simulink model "untitled1"  (R2012b)
settings: Solver=ode45  StartTime=0.0  StopTime=10.0  RelTol=1e-9
settings Model: Creator=Katarina  LastModifiedBy=Katarina
settings DataIOCC: LimitDataPoints=off
settings DebuggingCC: SolverPrmCheckMsg=none

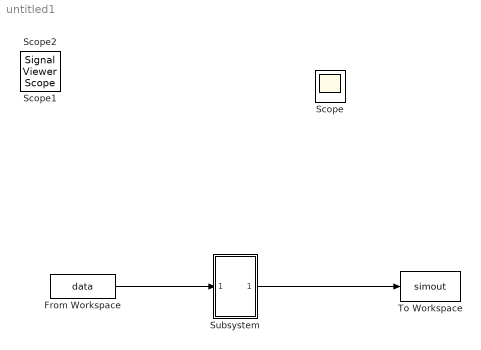
== system untitled1 ==
  From Workspace : FromWorkspace  VariableName=data  SampleTime=0
  Scope : Scope
  Subsystem : Subsystem
  To Workspace : ToWorkspace  VariableName=simout  SampleTime=-1  SaveFormat=Timeseries
  Scope1 : SignalViewerScope  IOType=viewer  RefreshTime=0.035000
  Scope2 : SignalViewerScope  IOType=viewer  RefreshTime=0.035000
  wires:
  Subsystem/1(Out1) -> To Workspace/1
  From Workspace/1 -> Subsystem/1(In1)

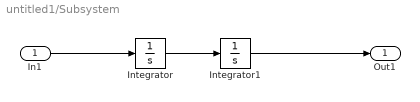
== system untitled1/Subsystem ==
  In1 : Inport
  Integrator : Integrator
  Integrator1 : Integrator
  Out1 : Outport
  wires:
  Integrator1/1 -> Out1/1
  Integrator/1 -> Integrator1/1
  In1/1 -> Integrator/1
